simulink model "simulinkexp1"  (R2018a)
settings: Solver=VariableStepAuto  StartTime=0.0  StopTime=tmax  RelTol=1e-3
values from neighbouring files (symbols this model uses):
  L1 = str2double(get(handles.L1,'String'))    [guigui.m]
  L2 = str2double(get(handles.L2,'String'))    [guigui.m]
  w0 = str2double(get(handles.w0,'String'))    [guigui.m]
libraries: vrlib x6
settings Model: Creator=yoors  LastModifiedBy=yoors

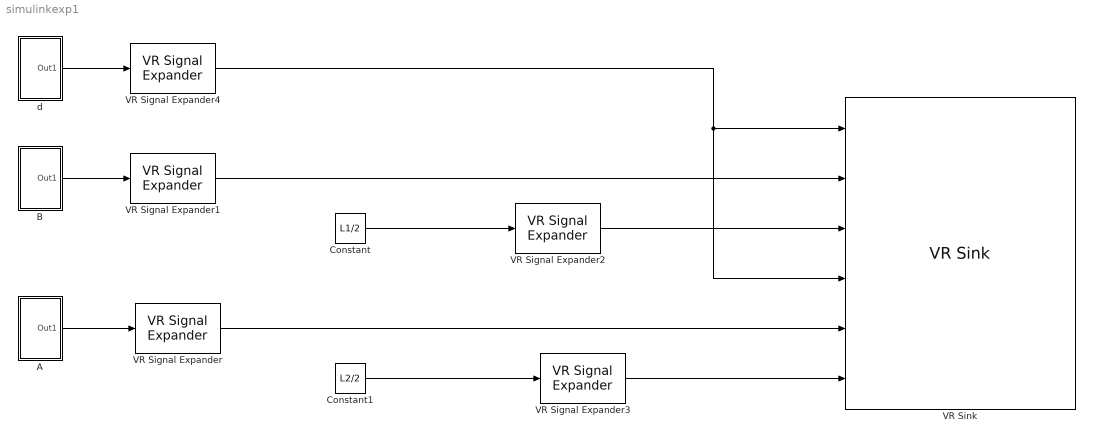
== system simulinkexp1 ==
  A : Subsystem
  B : Subsystem
  Constant : Constant  Value=L1/2
  Constant1 : Constant  Value=L2/2
  VR Signal Expander : vrlib/VR Signal Expander  outwidth=4  outidx=[4]
      settings: SourceProductName=Simulink 3D Animation  SourceProductBaseCode=VR
  VR Signal Expander1 : vrlib/VR Signal Expander  outwidth=4  outidx=[4]
      settings: SourceProductName=Simulink 3D Animation  SourceProductBaseCode=VR
  VR Signal Expander2 : vrlib/VR Signal Expander  outwidth=3  outidx=[2]
      settings: SourceProductName=Simulink 3D Animation  SourceProductBaseCode=VR
  VR Signal Expander3 : vrlib/VR Signal Expander  outwidth=3  outidx=[2]
      settings: SourceProductName=Simulink 3D Animation  SourceProductBaseCode=VR
  VR Signal Expander4 : vrlib/VR Signal Expander  outwidth=3  outidx=[2]
      settings: SourceProductName=Simulink 3D Animation  SourceProductBaseCode=VR
  VR Sink : vrlib/VR Sink  InstantiateOnLoad=on  SampleTime=0.1  ViewEnable=on  RemoteChange=off  RemoteView=off  FieldsWritten=piston.translation.3.1.1.double#L1.rotation.4.1.1.double#L1.scale.3.1.1.double#L1.translation.3.1.1.double#L2.rotation.4.1.1.double#L2.scale.3.1.1.double  WorldFileName=vrml1.wrl  AutoView=off  VideoDimensions=[]  AllowVariableSize=off
      settings: SourceProductBaseCode=VR
  d : Subsystem
  wires:
  A/1(Out1) -> VR Signal Expander/1
  B/1(Out1) -> VR Signal Expander1/1
  d/1(Out1) -> VR Signal Expander4/1
  VR Signal Expander4/1 -> VR Sink/4, VR Sink/1
  VR Signal Expander1/1 -> VR Sink/2
  VR Signal Expander/1 -> VR Sink/5
  Constant/1 -> VR Signal Expander2/1
  Constant1/1 -> VR Signal Expander3/1
  VR Signal Expander2/1 -> VR Sink/3
  VR Signal Expander3/1 -> VR Sink/6

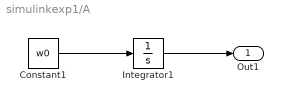
== system simulinkexp1/A ==
  Constant1 : Constant  Value=w0
  Integrator1 : Integrator
  Out1 : Outport
  wires:
  Constant1/1 -> Integrator1/1
  Integrator1/1 -> Out1/1

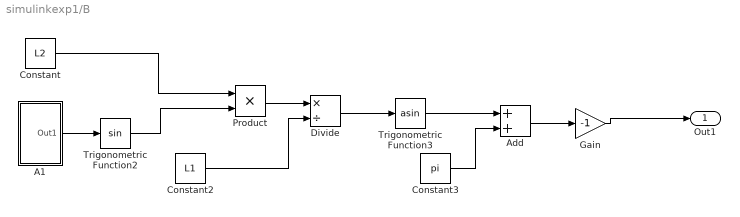
== system simulinkexp1/B ==
  A1 : Subsystem
  Add : Sum
  Constant : Constant  Value=L2
  Constant2 : Constant  Value=L1
  Constant3 : Constant  Value=pi
  Divide : Product  Inputs=*/
  Gain : Gain  Gain=-1
  Product : Product
  Trigonometric Function2 : Trigonometry
  Trigonometric Function3 : Trigonometry  Operator=asin
  Out1 : Outport
  wires:
  Trigonometric Function2/1 -> Product/2
  Constant3/1 -> Add/2
  Constant/1 -> Product/1
  Divide/1 -> Trigonometric Function3/1
  Product/1 -> Divide/1
  Trigonometric Function3/1 -> Add/1
  Constant2/1 -> Divide/2
  A1/1(Out1) -> Trigonometric Function2/1
  Add/1 -> Gain/1
  Gain/1 -> Out1/1

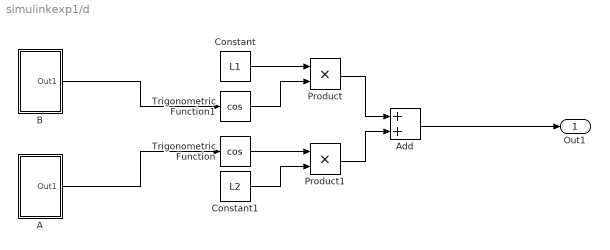
== system simulinkexp1/d ==
  A : Subsystem
  Add : Sum
  B : Subsystem
  Constant : Constant  Value=L1
  Constant1 : Constant  Value=L2
  Product : Product
  Product1 : Product
  Trigonometric Function : Trigonometry  Operator=cos
  Trigonometric Function1 : Trigonometry  Operator=cos
  Out1 : Outport
  wires:
  B/1(Out1) -> Trigonometric Function1/1
  Trigonometric Function1/1 -> Product/2
  Product/1 -> Add/1
  Trigonometric Function/1 -> Product1/1
  Constant/1 -> Product/1
  Constant1/1 -> Product1/2
  Product1/1 -> Add/2
  A/1(Out1) -> Trigonometric Function/1
  Add/1 -> Out1/1

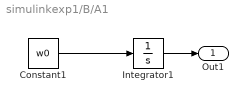
== system simulinkexp1/B/A1 ==
  Constant1 : Constant  Value=w0
  Integrator1 : Integrator
  Out1 : Outport
  wires:
  Constant1/1 -> Integrator1/1
  Integrator1/1 -> Out1/1

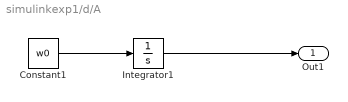
== system simulinkexp1/d/A ==
  Constant1 : Constant  Value=w0
  Integrator1 : Integrator
  Out1 : Outport
  wires:
  Constant1/1 -> Integrator1/1
  Integrator1/1 -> Out1/1

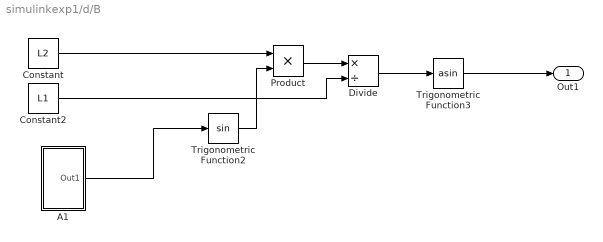
== system simulinkexp1/d/B ==
  A1 : Subsystem
  Constant : Constant  Value=L2
  Constant2 : Constant  Value=L1
  Divide : Product  Inputs=*/
  Product : Product
  Trigonometric Function2 : Trigonometry
  Trigonometric Function3 : Trigonometry  Operator=asin
  Out1 : Outport
  wires:
  Trigonometric Function2/1 -> Product/2
  Constant/1 -> Product/1
  Divide/1 -> Trigonometric Function3/1
  Product/1 -> Divide/1
  Constant2/1 -> Divide/2
  A1/1(Out1) -> Trigonometric Function2/1
  Trigonometric Function3/1 -> Out1/1

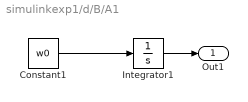
== system simulinkexp1/d/B/A1 ==
  Constant1 : Constant  Value=w0
  Integrator1 : Integrator
  Out1 : Outport
  wires:
  Constant1/1 -> Integrator1/1
  Integrator1/1 -> Out1/1
